simulink model "Data_Center_24hr_Total_Power_Analysis_Ref83_Simulation"  (R2024b)
settings: Solver=ode45  StartTime=0.0  StopTime=24  RelTol=1e-4
InitFcn:
  | load('DataCenterPower.mat')
libraries: spsThreePhaseSeriesRLCBranchLib x8, spsThreePhaseParallelRLCLoadLib x7, spsThreePhaseDynamicLoadLib x7, spsGroundLib x4, spsThreePhaseProgrammableVoltageSourceLib x2, spsThreePhaseTransformerTwoWindingsLib x2, spsThreePhaseBreakerLib x2, spsPower3phInstantaneousLib x1, spsThreePhaseVIMeasurementLib x1, sps_lib x1
settings Model: Creator=Kapla  LastModifiedBy=Kapla
settings DataIOCC: SaveFormat=Array  SaveOutput=off  SaveTime=off  ReturnWorkspaceOutputs=off
settings DebuggingCC: SaveWithParameterizedLinksMsg=none  IgnoredZcDiagnostic=none  StateNameClashWarn=warning  ArithmeticOperatorsInVariantConditions=warning
settings GRTTargetCC: TargetLangStandard=C89/C90 (ANSI)

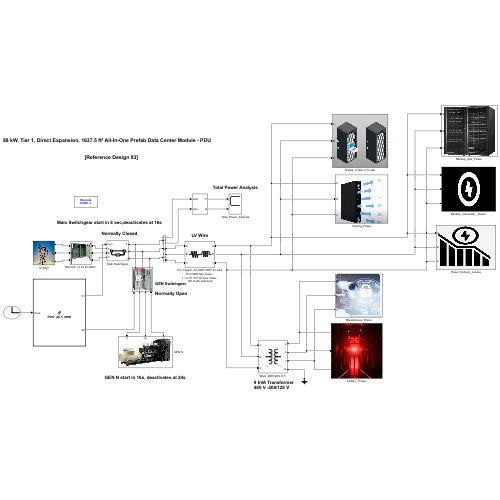
[thumbnail: Simulink's stored preview of the top-level diagram]
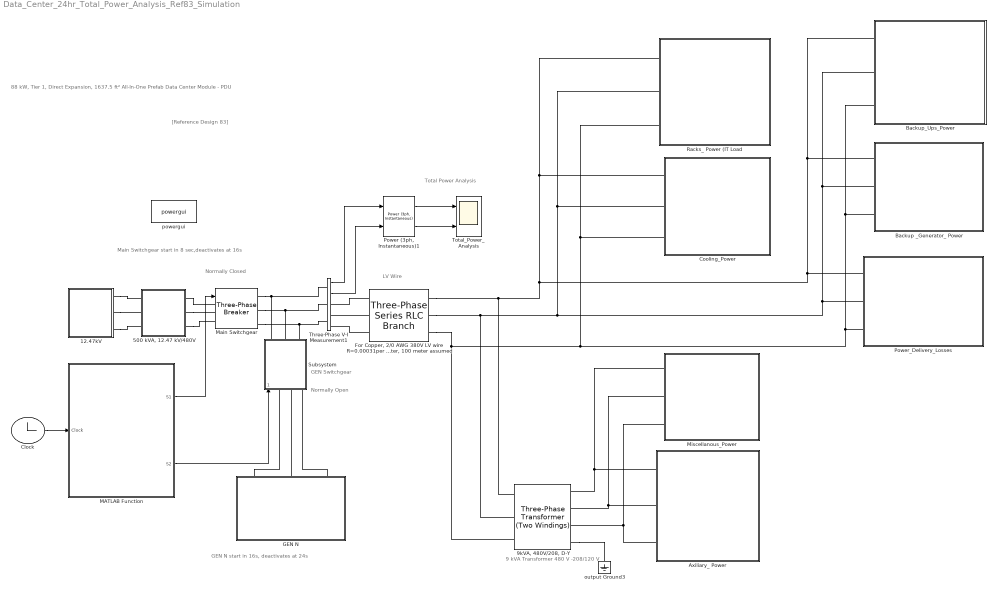
== system Data_Center_24hr_Total_Power_Analysis_Ref83_Simulation ==
  note: LV Wire
  note: Normally Open
  note: Normally Closed
  note: Main Switchgear start in 8 sec,deactivates at 16s
  note: GEN N start in 16s, deactivates at 24s
  note: GEN Switchgear
  note: [Reference Design 83]
  note: 88 kW, Tier 1, Direct Expansion, 1637.5 ft² All-In-One Prefab Data Center Module - PDU
  note: 9 kVA Transformer
      | 480 V -208/120 V
  note: Total Power Analysis
  12.47kV : Subsystem
      mask Display: image('Power_Grid_.png');
  "500 kVA, 12.47 kV/480V " : Subsystem
      mask Display: image('Data_Center_Transformer_Tier_1.png');
  "9kVA, 480V/208, D-Y" : spsThreePhaseTransformerTwoWindingsLib/Three-Phase Transformer (Two Windings)  Winding1Connection=Yg  Winding2Connection=Yn  CoreType=Three single-phase transformers  SetSaturation=off  Hysteresis=off  DataFile='hysteresis'  SetInitialFlux=off  Measurements=None  UNITS=pu  NominalPower=[ 9e3 , 60 ]  Winding1=[ 480 , 0.002 , 0.08 ]  Winding2=[ 208 , 0.002 , 0.08 ]  Rm=500  Lm=500  L0=0.5  Saturation=[ 0,0 ; 0.0024,1.2 ; 1.0,1.52 ]  InitialFluxes=[ 0.8 , -0.8 , 0.7 ]  BreakLoop=off  DiscreteSolver=Trapezoidal iterative  DataType=off  TransfoNumber=1
  Axiliary_ Power : Subsystem
      mask Display: image('Lighting_monitoring.png');
  "Backup _Generator_ Power " : Subsystem
      mask Display: image('back up_generator_power.png');
  "Backup_Ups_Power " : Subsystem
      mask Display: image('UPS.png');
  Clock : Clock
  Cooling_Power : Subsystem
      mask Display: image('Coolin.png');
  "For Copper, 2/0 AWG 380V LV wire R=0.00031per meter, L = 0.15 *10^-6 H per meter, 100 meter assumed " : spsThreePhaseSeriesRLCBranchLib/Three-Phase Series RLC Branch  LConnTagsString=A|B|C  RConnTagsString=A|B|C  BranchType=RL  Resistance=0.00031*100  Inductance=0.15e-6*100  Capacitance=[]  Measurements=None
  GEN N : Subsystem
      mask Display: image('Back_up_Generator.png');
  MATLAB Function : MATLAB Function  TreatAsAtomicUnit=on
  Main Switchgear : spsThreePhaseBreakerLib/Three-Phase Breaker  InitialState=closed  SwitchA=on  SwitchB=on  SwitchC=on  SwitchTimes="[8  16]"  External=on  BreakerResistance=10  SnubberResistance=1e-6  SnubberCapacitance=inf  Measurements=None
  Miscellanous_Power : Subsystem
      mask Display: image('Data_Center_Security.png');
  "Power (3ph, Instantaneous)1" : spsPower3phInstantaneousLib/Power (3ph, Instantaneous)
  Power_Delivery_Losses : Subsystem
      mask Display: image('Power_Delivery_losses.png');
  Racks_ Power (IT Load : Subsystem
      mask Display: image('racks_server.png');
  Subsystem : Subsystem
      mask Display: image('GEN_Switch_gear_500kW.png');
  Three-Phase V-I Measurement1 : spsThreePhaseVIMeasurementLib/Three-Phase V-I Measurement  VoltageMeasurement=phase-to-ground  SetLabelV=off  LabelV=V1  Vpu=off  VpuLL=off  CurrentMeasurement=yes  SetLabelI=off  LabelI=I1  Ipu=off  Pbase=100e6  Vbase=500e3  OutputType=Magnitude  PhasorSimulation=off  PSBequivalent=0
  Total_Power_Analysis : Scope  NumInputPorts=2
  output Ground3 : spsGroundLib/Ground  LConnTagsString=a
  powergui : sps_lib/powergui  Priority=1  SimulationMode=Discrete  SampleTime=100e-6  frequency=60  Iterations=50  frequencyindice=60  Pbase=100e6  ErrMax=1e-4  UnitsV=kV  UnitsW=MW  buscounter=0  FunctionMessages=off  echomessages=off  EnableUseOfTLC=off  CurrentSourceSwitches=off  DisableSnubberDevices=off  DisableRonSwitches=off  DisableVfSwitches=off  DisplayEquations=off  AutomaticDiscreteSolvers=off  SolverType=Tustin/Backward Euler (TBE)  Interpol=off  ExternalGateDelay=off  methode=off  Ts=100  x0status=blocks  SPID=on  SwTol=0  HookPort=off  NonlinearTolerance=1e-4  nMaxIteration=100  ContinueOnMaxIteration=off  RestoreLinks=warning  ResistiveCurrentMeasurement=off  Frange=[0:2:500]  Ylog=off  Xlog=on  ShowGrid=off  save=off  variable=ZData  structure=0  ZoomFFT=off  StartTime=0.0  cycles=1  DisplayStyle=1  fundamental=60  FreqAxis=off  MaxFrequency=1000  frequencyindicesteady=1  RmsSteady=1  display=off
  wires:
  Three-Phase V-I Measurement1/2 -> "Power (3ph, Instantaneous)1"/2
  Three-Phase V-I Measurement1/1 -> "Power (3ph, Instantaneous)1"/1
  MATLAB Function/1(S1) -> Main Switchgear/1
  Clock/1 -> MATLAB Function/1(Clock)
  "Power (3ph, Instantaneous)1"/1 -> Total_Power_Analysis/1
  "Power (3ph, Instantaneous)1"/2 -> Total_Power_Analysis/2
  MATLAB Function/2(S2) -> Subsystem/1(com)
  connections:
  Power_Delivery_Losses/LConn3 -- "9kVA, 480V/208, D-Y"/LConn3 -- "For Copper, 2/0 AWG 380V LV wire R=0.00031per meter, L = 0.15 *10^-6 H per meter, 100 meter assumed "/RConn3 -- Racks_ Power (IT Load/LConn3 -- Cooling_Power/LConn3 -- "Backup _Generator_ Power "/LConn3 -- "Backup_Ups_Power "/LConn3
  Power_Delivery_Losses/LConn2 -- "9kVA, 480V/208, D-Y"/LConn2 -- "For Copper, 2/0 AWG 380V LV wire R=0.00031per meter, L = 0.15 *10^-6 H per meter, 100 meter assumed "/RConn2 -- Racks_ Power (IT Load/LConn2 -- Cooling_Power/LConn2 -- "Backup _Generator_ Power "/LConn2 -- "Backup_Ups_Power "/LConn2
  Cooling_Power/LConn1 -- Racks_ Power (IT Load/LConn1 -- "9kVA, 480V/208, D-Y"/LConn1 -- "For Copper, 2/0 AWG 380V LV wire R=0.00031per meter, L = 0.15 *10^-6 H per meter, 100 meter assumed "/RConn1 -- "Backup_Ups_Power "/LConn1 -- "Backup _Generator_ Power "/LConn1 -- Power_Delivery_Losses/LConn1
  Axiliary_ Power/LConn1 -- Miscellanous_Power/LConn1 -- "9kVA, 480V/208, D-Y"/RConn1
  Axiliary_ Power/LConn3 -- Miscellanous_Power/LConn3 -- "9kVA, 480V/208, D-Y"/RConn3
  Axiliary_ Power/LConn2 -- Miscellanous_Power/LConn2 -- "9kVA, 480V/208, D-Y"/RConn2
  "9kVA, 480V/208, D-Y"/RConn4 -- output Ground3/LConn1
  Main Switchgear/RConn1 -- Subsystem/RConn1 -- Three-Phase V-I Measurement1/LConn1
  Main Switchgear/RConn2 -- Subsystem/RConn2 -- Three-Phase V-I Measurement1/LConn2
  Main Switchgear/RConn3 -- Subsystem/RConn3 -- Three-Phase V-I Measurement1/LConn3
  12.47kV/RConn1 -- "500 kVA, 12.47 kV/480V "/LConn1
  "500 kVA, 12.47 kV/480V "/RConn1 -- Main Switchgear/LConn1
  "500 kVA, 12.47 kV/480V "/RConn2 -- Main Switchgear/LConn2
  12.47kV/RConn2 -- "500 kVA, 12.47 kV/480V "/LConn2
  "500 kVA, 12.47 kV/480V "/RConn3 -- Main Switchgear/LConn3
  12.47kV/RConn3 -- "500 kVA, 12.47 kV/480V "/LConn3
  GEN N/RConn1 -- Subsystem/LConn1
  GEN N/RConn2 -- Subsystem/LConn2
  GEN N/RConn3 -- Subsystem/LConn3
  "For Copper, 2/0 AWG 380V LV wire R=0.00031per meter, L = 0.15 *10^-6 H per meter, 100 meter assumed "/LConn1 -- Three-Phase V-I Measurement1/RConn1
  "For Copper, 2/0 AWG 380V LV wire R=0.00031per meter, L = 0.15 *10^-6 H per meter, 100 meter assumed "/LConn2 -- Three-Phase V-I Measurement1/RConn2
  "For Copper, 2/0 AWG 380V LV wire R=0.00031per meter, L = 0.15 *10^-6 H per meter, 100 meter assumed "/LConn3 -- Three-Phase V-I Measurement1/RConn3

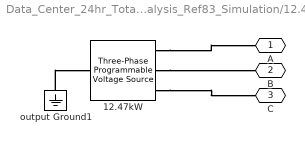
== system Data_Center_24hr_Total_Power_Analysis_Ref83_Simulation/12.47kV ==
  12.47kW : spsThreePhaseProgrammableVoltageSourceLib/Three-Phase Programmable Voltage Source  PositiveSequence="[12.47e3  0 60]"  VariationEntity=None  VariationType=Step  VariationTypeAlt=Step  VariationStep=-0.5  VariationRate=10  VariationMagnitude=0.5  VariationFrequency=1  VariationTiming=[0.2 1.2]  VariationPhaseA=off  Amplitudes=[1 0.8 1.2 1.0]  TimeValues=[0 0.1 0.15 0.2]  HarmonicGeneration=off  HarmonicA=[3 0.2 -25 0]  HarmonicB="[2 0.15  35 2]"  Timing="[0.05  3]"  BusType=swing  Pref=0  Qref=0  Qmin=-inf  Qmax=inf
  output Ground1 : spsGroundLib/Ground  LConnTagsString=a
  A : PMIOPort  Side=Right
  B : PMIOPort  Port=2  Side=Right
  C : PMIOPort  Port=3  Side=Right
  connections:
  output Ground1/LConn1 -- 12.47kW/LConn1
  12.47kW/RConn2 -- B/RConn1
  12.47kW/RConn3 -- C/RConn1
  12.47kW/RConn1 -- A/RConn1

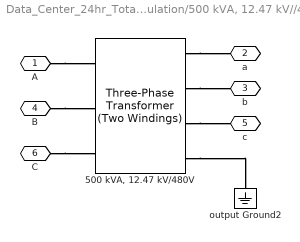
== system Data_Center_24hr_Total_Power_Analysis_Ref83_Simulation/500 kVA, 12.47 kV//480V  ==
  "500 kVA, 12.47 kV/480V " : spsThreePhaseTransformerTwoWindingsLib/Three-Phase Transformer (Two Windings)  Winding1Connection=Yg  Winding2Connection=Yn  CoreType=Three single-phase transformers  SetSaturation=off  Hysteresis=off  DataFile='hysteresis'  SetInitialFlux=off  Measurements=None  UNITS=pu  NominalPower=[ 500e3 , 60 ]  Winding1=[ 12.47e3 , 0.002 , 0.08 ]  Winding2=[ 480 , 0.002 , 0.08 ]  Rm=500  Lm=500  L0=0.5  Saturation=[ 0,0 ; 0.0024,1.2 ; 1.0,1.52 ]  InitialFluxes=[ 0.8 , -0.8 , 0.7 ]  BreakLoop=off  DiscreteSolver=Trapezoidal iterative  DataType=off  TransfoNumber=1
  output Ground2 : spsGroundLib/Ground  LConnTagsString=a
  A : PMIOPort  Side=Left
  a : PMIOPort  Port=2  Side=Right
  b : PMIOPort  Port=3  Side=Right
  B : PMIOPort  Port=4  Side=Left
  c : PMIOPort  Port=5  Side=Right
  C : PMIOPort  Port=6  Side=Left
  connections:
  "500 kVA, 12.47 kV/480V "/RConn4 -- output Ground2/LConn1
  C/RConn1 -- "500 kVA, 12.47 kV/480V "/LConn3
  A/RConn1 -- "500 kVA, 12.47 kV/480V "/LConn1
  "500 kVA, 12.47 kV/480V "/RConn3 -- c/RConn1
  B/RConn1 -- "500 kVA, 12.47 kV/480V "/LConn2
  "500 kVA, 12.47 kV/480V "/RConn1 -- a/RConn1
  "500 kVA, 12.47 kV/480V "/RConn2 -- b/RConn1

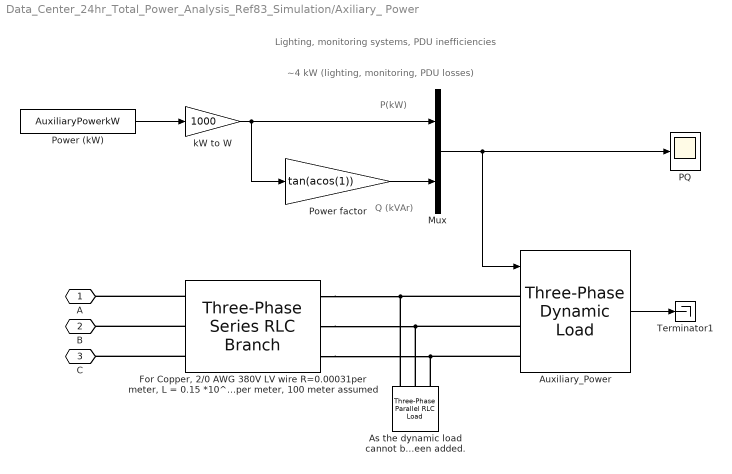
== system Data_Center_24hr_Total_Power_Analysis_Ref83_Simulation/Axiliary_ Power ==
  note: Q (kVAr)
  note: P(kW)
  note: ~4 kW (lighting, monitoring, PDU losses)
  note: Lighting, monitoring systems, PDU inefficiencies
  "As the dynamic load cannot be connected to an inductive network (R-L in series), a small resistive load (1 W) has been added." : spsThreePhaseParallelRLCLoadLib/Three-Phase Parallel RLC Load  LConnTagsString=A|B|C  Configuration=Y (grounded)  NominalVoltage=480  Vabc=[1e3 1e3 1e3]  Vabcp=[1e3 1e3 1e3]  NominalFrequency=60  UnbalancedPower=off  ActivePower=1  InductivePower=0  CapacitivePower=0  Pabc=[10e3 9e3 11e3]  QLabc=[100 90 110]  QCabc=[100 90 110]  Pabcp=[10e3 9e3 11e3]  QLabcp=[100 90 110]  QCabcp=[100 90 110]  Measurements=None  LoadType=constant Z
  Auxiliary_Power : spsThreePhaseDynamicLoadLib/Three-Phase Dynamic Load  NominalVoltage=[ 480 60 ]  ActiveReactivePowers=[3982 0*3982]  PositiveSequence=[1 -1.41063]  ExternalControl=on  NpNq="[1  1]"  TimeConstants="[0  0  0  0]"  MinimumVoltage=0.7  Tfilter=1e-4  LoadFlowParameters=[4 50000000 0 0 25000000]
  "For Copper, 2/0 AWG 380V LV wire R=0.00031per meter, L = 0.15 *10^-6 H per meter, 100 meter assumed " : spsThreePhaseSeriesRLCBranchLib/Three-Phase Series RLC Branch  LConnTagsString=A|B|C  RConnTagsString=A|B|C  BranchType=RL  Resistance=0.00031*100  Inductance=0.15e-6*100  Capacitance=[]  Measurements=None
  Mux : Mux  Inputs=2
  PQ : Scope
  Power (kW) : FromWorkspace  VariableName=AuxiliaryPowerkW
  Power factor : Gain  Gain=tan(acos(1))
  Terminator1 : Terminator
  kW to W : Gain  Gain=1000
  A : PMIOPort  Side=Left
  B : PMIOPort  Port=2  Side=Left
  C : PMIOPort  Port=3  Side=Left
  wires:
  Auxiliary_Power/1 -> Terminator1/1
  Power (kW)/1 -> kW to W/1
  kW to W/1 -> Power factor/1, Mux/1
  Power factor/1 -> Mux/2
  Mux/1 -> PQ/1, Auxiliary_Power/1
  connections:
  "For Copper, 2/0 AWG 380V LV wire R=0.00031per meter, L = 0.15 *10^-6 H per meter, 100 meter assumed "/LConn2 -- B/RConn1
  "For Copper, 2/0 AWG 380V LV wire R=0.00031per meter, L = 0.15 *10^-6 H per meter, 100 meter assumed "/LConn1 -- A/RConn1
  "For Copper, 2/0 AWG 380V LV wire R=0.00031per meter, L = 0.15 *10^-6 H per meter, 100 meter assumed "/LConn3 -- C/RConn1
  "For Copper, 2/0 AWG 380V LV wire R=0.00031per meter, L = 0.15 *10^-6 H per meter, 100 meter assumed "/RConn1 -- Auxiliary_Power/LConn1 -- "As the dynamic load cannot be connected to an inductive network (R-L in series), a small resistive load (1 W) has been added."/LConn1
  "For Copper, 2/0 AWG 380V LV wire R=0.00031per meter, L = 0.15 *10^-6 H per meter, 100 meter assumed "/RConn2 -- Auxiliary_Power/LConn2 -- "As the dynamic load cannot be connected to an inductive network (R-L in series), a small resistive load (1 W) has been added."/LConn2
  "For Copper, 2/0 AWG 380V LV wire R=0.00031per meter, L = 0.15 *10^-6 H per meter, 100 meter assumed "/RConn3 -- Auxiliary_Power/LConn3 -- "As the dynamic load cannot be connected to an inductive network (R-L in series), a small resistive load (1 W) has been added."/LConn3

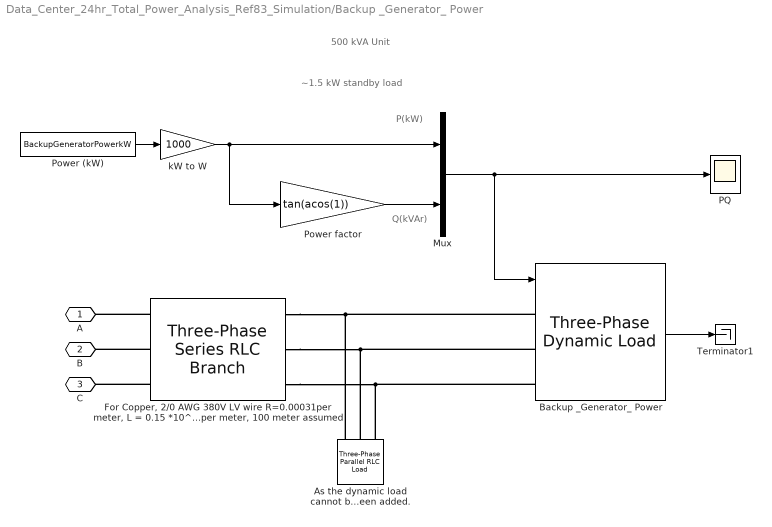
== system Data_Center_24hr_Total_Power_Analysis_Ref83_Simulation/Backup _Generator_ Power  ==
  note: Q(kVAr)
  note: P(kW)
  note: 500 kVA Unit
      |
      | ​
  note: ~1.5 kW standby load
      |
      | ​
  "As the dynamic load cannot be connected to an inductive network (R-L in series), a small resistive load (1 W) has been added." : spsThreePhaseParallelRLCLoadLib/Three-Phase Parallel RLC Load  LConnTagsString=A|B|C  Configuration=Y (grounded)  NominalVoltage=480  Vabc=[1e3 1e3 1e3]  Vabcp=[1e3 1e3 1e3]  NominalFrequency=60  UnbalancedPower=off  ActivePower=1  InductivePower=0  CapacitivePower=0  Pabc=[10e3 9e3 11e3]  QLabc=[100 90 110]  QCabc=[100 90 110]  Pabcp=[10e3 9e3 11e3]  QLabcp=[100 90 110]  QCabcp=[100 90 110]  Measurements=None  LoadType=constant Z
  "Backup _Generator_ Power " : spsThreePhaseDynamicLoadLib/Three-Phase Dynamic Load  NominalVoltage=[ 480 60 ]  ActiveReactivePowers=[1658 0*1658]  PositiveSequence=[1 -1.41063]  ExternalControl=on  NpNq="[1  1]"  TimeConstants="[0  0  0  0]"  MinimumVoltage=0.7  Tfilter=1e-4  LoadFlowParameters=[4 50000000 0 0 25000000]
  "For Copper, 2/0 AWG 380V LV wire R=0.00031per meter, L = 0.15 *10^-6 H per meter, 100 meter assumed " : spsThreePhaseSeriesRLCBranchLib/Three-Phase Series RLC Branch  LConnTagsString=A|B|C  RConnTagsString=A|B|C  BranchType=RL  Resistance=0.00031*100  Inductance=0.15e-6*100  Capacitance=[]  Measurements=None
  Mux : Mux  Inputs=2
  PQ : Scope
  Power (kW) : FromWorkspace  VariableName=BackupGeneratorPowerkW
  Power factor : Gain  Gain=tan(acos(1))
  Terminator1 : Terminator
  kW to W : Gain  Gain=1000
  A : PMIOPort  Side=Left
  B : PMIOPort  Port=2  Side=Left
  C : PMIOPort  Port=3  Side=Left
  wires:
  Power (kW)/1 -> kW to W/1
  "Backup _Generator_ Power "/1 -> Terminator1/1
  kW to W/1 -> Power factor/1, Mux/1
  Power factor/1 -> Mux/2
  Mux/1 -> PQ/1, "Backup _Generator_ Power "/1
  connections:
  "For Copper, 2/0 AWG 380V LV wire R=0.00031per meter, L = 0.15 *10^-6 H per meter, 100 meter assumed "/RConn3 -- "As the dynamic load cannot be connected to an inductive network (R-L in series), a small resistive load (1 W) has been added."/LConn3 -- "Backup _Generator_ Power "/LConn3
  "For Copper, 2/0 AWG 380V LV wire R=0.00031per meter, L = 0.15 *10^-6 H per meter, 100 meter assumed "/RConn1 -- "As the dynamic load cannot be connected to an inductive network (R-L in series), a small resistive load (1 W) has been added."/LConn1 -- "Backup _Generator_ Power "/LConn1
  "For Copper, 2/0 AWG 380V LV wire R=0.00031per meter, L = 0.15 *10^-6 H per meter, 100 meter assumed "/RConn2 -- "As the dynamic load cannot be connected to an inductive network (R-L in series), a small resistive load (1 W) has been added."/LConn2 -- "Backup _Generator_ Power "/LConn2
  "For Copper, 2/0 AWG 380V LV wire R=0.00031per meter, L = 0.15 *10^-6 H per meter, 100 meter assumed "/LConn2 -- B/RConn1
  "For Copper, 2/0 AWG 380V LV wire R=0.00031per meter, L = 0.15 *10^-6 H per meter, 100 meter assumed "/LConn3 -- C/RConn1
  "For Copper, 2/0 AWG 380V LV wire R=0.00031per meter, L = 0.15 *10^-6 H per meter, 100 meter assumed "/LConn1 -- A/RConn1

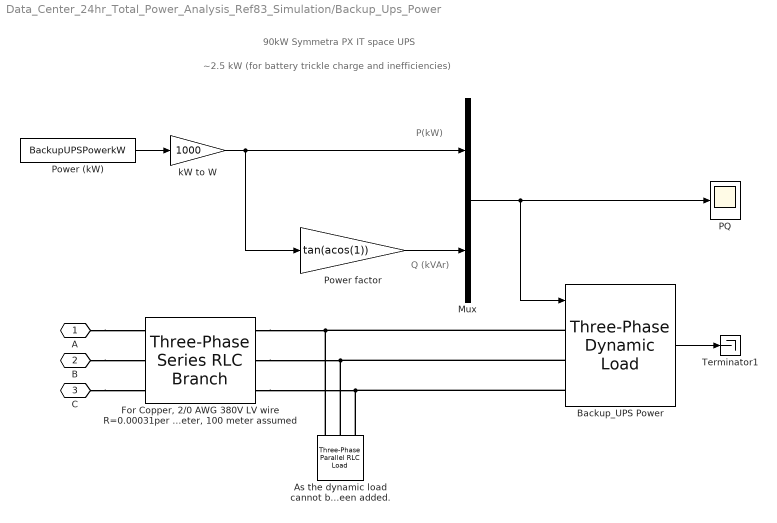
== system Data_Center_24hr_Total_Power_Analysis_Ref83_Simulation/Backup_Ups_Power  ==
  note: Q (kVAr)
  note: P(kW)
  note: ~2.5 kW (for battery trickle charge and inefficiencies)
  note: 90kW Symmetra PX IT space UPS
      |
      | ​
  "As the dynamic load cannot be connected to an inductive network (R-L in series), a small resistive load (1 W) has been added." : spsThreePhaseParallelRLCLoadLib/Three-Phase Parallel RLC Load  LConnTagsString=A|B|C  Configuration=Y (grounded)  NominalVoltage=480  Vabc=[1e3 1e3 1e3]  Vabcp=[1e3 1e3 1e3]  NominalFrequency=60  UnbalancedPower=off  ActivePower=1  InductivePower=0  CapacitivePower=0  Pabc=[10e3 9e3 11e3]  QLabc=[100 90 110]  QCabc=[100 90 110]  Pabcp=[10e3 9e3 11e3]  QLabcp=[100 90 110]  QCabcp=[100 90 110]  Measurements=None  LoadType=constant Z
  Backup_UPS Power : spsThreePhaseDynamicLoadLib/Three-Phase Dynamic Load  NominalVoltage=[ 480 60 ]  ActiveReactivePowers=[2559 0*2559]  PositiveSequence=[1 -1.41063]  ExternalControl=on  NpNq="[1  1]"  TimeConstants="[0  0  0  0]"  MinimumVoltage=0.7  Tfilter=1e-4  LoadFlowParameters=[4 50000000 0 0 25000000]
  "For Copper, 2/0 AWG 380V LV wire R=0.00031per meter, L = 0.15 *10^-6 H per meter, 100 meter assumed " : spsThreePhaseSeriesRLCBranchLib/Three-Phase Series RLC Branch  LConnTagsString=A|B|C  RConnTagsString=A|B|C  BranchType=RL  Resistance=0.00031*100  Inductance=0.15e-6*100  Capacitance=[]  Measurements=None
  Mux : Mux  Inputs=2
  PQ : Scope
  Power (kW) : FromWorkspace  VariableName=BackupUPSPowerkW
  Power factor : Gain  Gain=tan(acos(1))
  Terminator1 : Terminator
  kW to W : Gain  Gain=1000
  A : PMIOPort  Side=Left
  B : PMIOPort  Port=2  Side=Left
  C : PMIOPort  Port=3  Side=Left
  wires:
  Power (kW)/1 -> kW to W/1
  kW to W/1 -> Power factor/1, Mux/1
  Backup_UPS Power/1 -> Terminator1/1
  Power factor/1 -> Mux/2
  Mux/1 -> PQ/1, Backup_UPS Power/1
  connections:
  A/RConn1 -- "For Copper, 2/0 AWG 380V LV wire R=0.00031per meter, L = 0.15 *10^-6 H per meter, 100 meter assumed "/LConn1
  C/RConn1 -- "For Copper, 2/0 AWG 380V LV wire R=0.00031per meter, L = 0.15 *10^-6 H per meter, 100 meter assumed "/LConn3
  B/RConn1 -- "For Copper, 2/0 AWG 380V LV wire R=0.00031per meter, L = 0.15 *10^-6 H per meter, 100 meter assumed "/LConn2
  "For Copper, 2/0 AWG 380V LV wire R=0.00031per meter, L = 0.15 *10^-6 H per meter, 100 meter assumed "/RConn1 -- Backup_UPS Power/LConn1 -- "As the dynamic load cannot be connected to an inductive network (R-L in series), a small resistive load (1 W) has been added."/LConn1
  "For Copper, 2/0 AWG 380V LV wire R=0.00031per meter, L = 0.15 *10^-6 H per meter, 100 meter assumed "/RConn2 -- Backup_UPS Power/LConn2 -- "As the dynamic load cannot be connected to an inductive network (R-L in series), a small resistive load (1 W) has been added."/LConn2
  "For Copper, 2/0 AWG 380V LV wire R=0.00031per meter, L = 0.15 *10^-6 H per meter, 100 meter assumed "/RConn3 -- Backup_UPS Power/LConn3 -- "As the dynamic load cannot be connected to an inductive network (R-L in series), a small resistive load (1 W) has been added."/LConn3

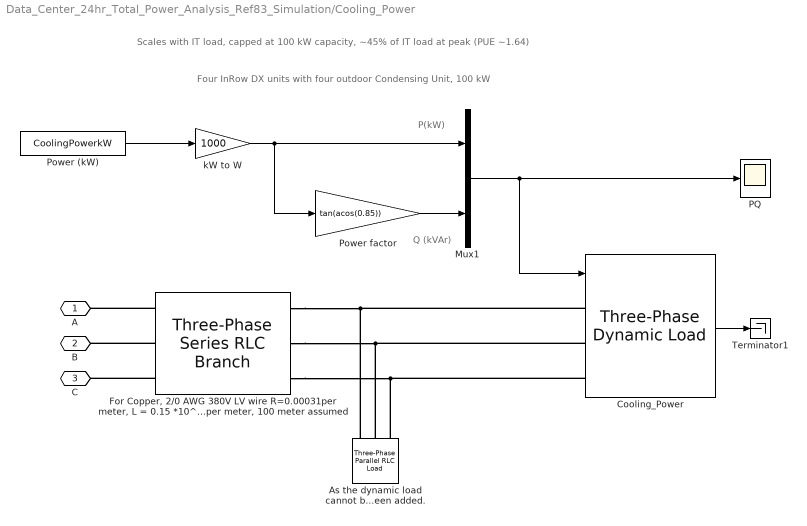
== system Data_Center_24hr_Total_Power_Analysis_Ref83_Simulation/Cooling_Power ==
  note: Q (kVAr)
  note: P(kW)
  note: Four InRow DX units with four outdoor Condensing Unit, 100 kW
  note: Scales with IT load, capped at 100 kW capacity, ~45% of IT load at peak (PUE ~1.64)
  "As the dynamic load cannot be connected to an inductive network (R-L in series), a small resistive load (1 W) has been added." : spsThreePhaseParallelRLCLoadLib/Three-Phase Parallel RLC Load  LConnTagsString=A|B|C  Configuration=Y (grounded)  NominalVoltage=480  Vabc=[1e3 1e3 1e3]  Vabcp=[1e3 1e3 1e3]  NominalFrequency=60  UnbalancedPower=off  ActivePower=1  InductivePower=0  CapacitivePower=0  Pabc=[10e3 9e3 11e3]  QLabc=[100 90 110]  QCabc=[100 90 110]  Pabcp=[10e3 9e3 11e3]  QLabcp=[100 90 110]  QCabcp=[100 90 110]  Measurements=None  LoadType=constant Z
  Cooling_Power : spsThreePhaseDynamicLoadLib/Three-Phase Dynamic Load  NominalVoltage=[ 480 60 ]  ActiveReactivePowers=[20378 0.61974*20378]  PositiveSequence=[1 -1.41063]  ExternalControl=on  NpNq="[1  1]"  TimeConstants="[0  0  0  0]"  MinimumVoltage=0.7  Tfilter=1e-4  LoadFlowParameters=[4 50000000 0 0 25000000]
  "For Copper, 2/0 AWG 380V LV wire R=0.00031per meter, L = 0.15 *10^-6 H per meter, 100 meter assumed " : spsThreePhaseSeriesRLCBranchLib/Three-Phase Series RLC Branch  LConnTagsString=A|B|C  RConnTagsString=A|B|C  BranchType=RL  Resistance=0.00031*100  Inductance=0.15e-6*100  Capacitance=[]  Measurements=None
  Mux1 : Mux  Inputs=2
  PQ : Scope
  Power (kW) : FromWorkspace  VariableName=CoolingPowerkW
  Power factor : Gain  Gain=tan(acos(0.85))
  Terminator1 : Terminator
  kW to W : Gain  Gain=1000
  A : PMIOPort  Side=Left
  B : PMIOPort  Port=2  Side=Left
  C : PMIOPort  Port=3  Side=Left
  wires:
  Power (kW)/1 -> kW to W/1
  Cooling_Power/1 -> Terminator1/1
  kW to W/1 -> Mux1/1, Power factor/1
  Power factor/1 -> Mux1/2
  Mux1/1 -> PQ/1, Cooling_Power/1
  connections:
  "For Copper, 2/0 AWG 380V LV wire R=0.00031per meter, L = 0.15 *10^-6 H per meter, 100 meter assumed "/LConn3 -- C/RConn1
  "For Copper, 2/0 AWG 380V LV wire R=0.00031per meter, L = 0.15 *10^-6 H per meter, 100 meter assumed "/LConn2 -- B/RConn1
  "For Copper, 2/0 AWG 380V LV wire R=0.00031per meter, L = 0.15 *10^-6 H per meter, 100 meter assumed "/LConn1 -- A/RConn1
  "For Copper, 2/0 AWG 380V LV wire R=0.00031per meter, L = 0.15 *10^-6 H per meter, 100 meter assumed "/RConn1 -- Cooling_Power/LConn1 -- "As the dynamic load cannot be connected to an inductive network (R-L in series), a small resistive load (1 W) has been added."/LConn1
  "For Copper, 2/0 AWG 380V LV wire R=0.00031per meter, L = 0.15 *10^-6 H per meter, 100 meter assumed "/RConn2 -- Cooling_Power/LConn2 -- "As the dynamic load cannot be connected to an inductive network (R-L in series), a small resistive load (1 W) has been added."/LConn2
  "For Copper, 2/0 AWG 380V LV wire R=0.00031per meter, L = 0.15 *10^-6 H per meter, 100 meter assumed "/RConn3 -- Cooling_Power/LConn3 -- "As the dynamic load cannot be connected to an inductive network (R-L in series), a small resistive load (1 W) has been added."/LConn3

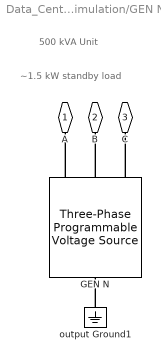
== system Data_Center_24hr_Total_Power_Analysis_Ref83_Simulation/GEN N ==
  note: ~1.5 kW standby load
      |
      | ​
  note: 500 kVA Unit
      |
      | ​
  GEN N : spsThreePhaseProgrammableVoltageSourceLib/Three-Phase Programmable Voltage Source  PositiveSequence="[480 0  60]"  VariationEntity=None  VariationType=Step  VariationTypeAlt=Step  VariationStep=-0.5  VariationRate=10  VariationMagnitude=0.5  VariationFrequency=1  VariationTiming=[0.2 1.2]  VariationPhaseA=off  Amplitudes=[1 0.8 1.2 1.0]  TimeValues=[0 0.1 0.15 0.2]  HarmonicGeneration=off  HarmonicA=[3 0.2 -25 0]  HarmonicB="[2 0.15  35 2]"  Timing="[0.05  3]"  BusType=PV  Pref=500e3  Qref=0  Qmin=-inf  Qmax=inf
  output Ground1 : spsGroundLib/Ground  LConnTagsString=a
  A : PMIOPort  Side=Right
  B : PMIOPort  Port=2  Side=Right
  C : PMIOPort  Port=3  Side=Right
  connections:
  GEN N/RConn2 -- B/RConn1
  output Ground1/LConn1 -- GEN N/LConn1
  GEN N/RConn1 -- A/RConn1
  GEN N/RConn3 -- C/RConn1

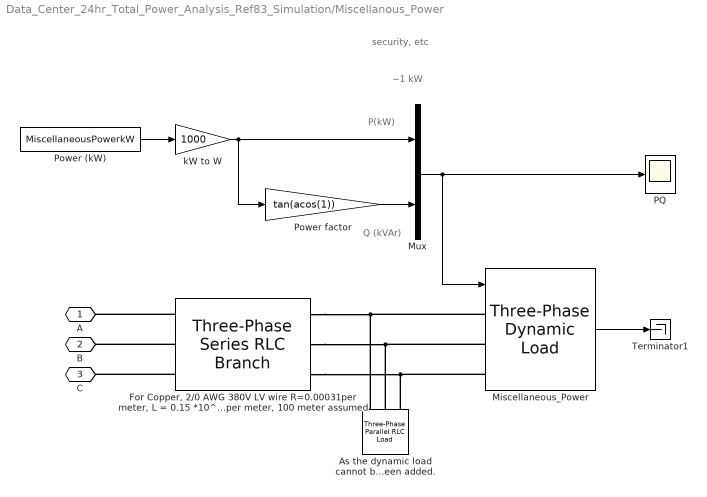
== system Data_Center_24hr_Total_Power_Analysis_Ref83_Simulation/Miscellanous_Power ==
  note: Q (kVAr)
  note: P(kW)
  note: security, etc
      |
      | ​
      |
      | ​
  note: ~1 kW
  "As the dynamic load cannot be connected to an inductive network (R-L in series), a small resistive load (1 W) has been added." : spsThreePhaseParallelRLCLoadLib/Three-Phase Parallel RLC Load  LConnTagsString=A|B|C  Configuration=Y (grounded)  NominalVoltage=480  Vabc=[1e3 1e3 1e3]  Vabcp=[1e3 1e3 1e3]  NominalFrequency=60  UnbalancedPower=off  ActivePower=1  InductivePower=0  CapacitivePower=0  Pabc=[10e3 9e3 11e3]  QLabc=[100 90 110]  QCabc=[100 90 110]  Pabcp=[10e3 9e3 11e3]  QLabcp=[100 90 110]  QCabcp=[100 90 110]  Measurements=None  LoadType=constant Z
  "For Copper, 2/0 AWG 380V LV wire R=0.00031per meter, L = 0.15 *10^-6 H per meter, 100 meter assumed " : spsThreePhaseSeriesRLCBranchLib/Three-Phase Series RLC Branch  LConnTagsString=A|B|C  RConnTagsString=A|B|C  BranchType=RL  Resistance=0.00031*100  Inductance=0.15e-6*100  Capacitance=[]  Measurements=None
  Miscellaneous_Power : spsThreePhaseDynamicLoadLib/Three-Phase Dynamic Load  NominalVoltage=[ 480 60 ]  ActiveReactivePowers=[1052 0*1052]  PositiveSequence=[1 -1.41063]  ExternalControl=on  NpNq="[1  1]"  TimeConstants="[0  0  0  0]"  MinimumVoltage=0.7  Tfilter=1e-4  LoadFlowParameters=[4 50000000 0 0 25000000]
  Mux : Mux  Inputs=2
  PQ : Scope
  Power (kW) : FromWorkspace  VariableName=MiscellaneousPowerkW
  Power factor : Gain  Gain=tan(acos(1))
  Terminator1 : Terminator
  kW to W : Gain  Gain=1000
  A : PMIOPort  Side=Left
  B : PMIOPort  Port=2  Side=Left
  C : PMIOPort  Port=3  Side=Left
  wires:
  Power (kW)/1 -> kW to W/1
  Miscellaneous_Power/1 -> Terminator1/1
  kW to W/1 -> Mux/1, Power factor/1
  Mux/1 -> PQ/1, Miscellaneous_Power/1
  Power factor/1 -> Mux/2
  connections:
  "For Copper, 2/0 AWG 380V LV wire R=0.00031per meter, L = 0.15 *10^-6 H per meter, 100 meter assumed "/LConn2 -- B/RConn1
  "For Copper, 2/0 AWG 380V LV wire R=0.00031per meter, L = 0.15 *10^-6 H per meter, 100 meter assumed "/LConn1 -- A/RConn1
  "For Copper, 2/0 AWG 380V LV wire R=0.00031per meter, L = 0.15 *10^-6 H per meter, 100 meter assumed "/LConn3 -- C/RConn1
  Miscellaneous_Power/LConn1 -- "For Copper, 2/0 AWG 380V LV wire R=0.00031per meter, L = 0.15 *10^-6 H per meter, 100 meter assumed "/RConn1 -- "As the dynamic load cannot be connected to an inductive network (R-L in series), a small resistive load (1 W) has been added."/LConn1
  Miscellaneous_Power/LConn2 -- "For Copper, 2/0 AWG 380V LV wire R=0.00031per meter, L = 0.15 *10^-6 H per meter, 100 meter assumed "/RConn2 -- "As the dynamic load cannot be connected to an inductive network (R-L in series), a small resistive load (1 W) has been added."/LConn2
  Miscellaneous_Power/LConn3 -- "For Copper, 2/0 AWG 380V LV wire R=0.00031per meter, L = 0.15 *10^-6 H per meter, 100 meter assumed "/RConn3 -- "As the dynamic load cannot be connected to an inductive network (R-L in series), a small resistive load (1 W) has been added."/LConn3

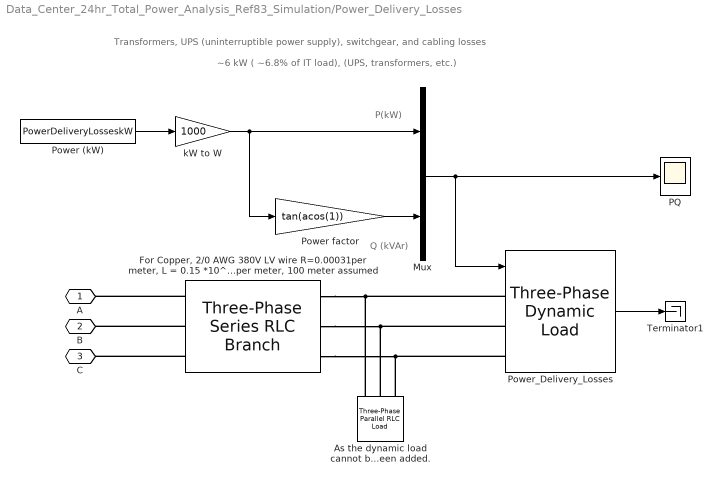
== system Data_Center_24hr_Total_Power_Analysis_Ref83_Simulation/Power_Delivery_Losses ==
  note: Q (kVAr)
  note: P(kW)
  note: ~6 kW ( ~6.8% of IT load), (UPS, transformers, etc.)
  note: Transformers, UPS (uninterruptible power supply), switchgear, and cabling losses
  "As the dynamic load cannot be connected to an inductive network (R-L in series), a small resistive load (1 W) has been added." : spsThreePhaseParallelRLCLoadLib/Three-Phase Parallel RLC Load  LConnTagsString=A|B|C  Configuration=Y (grounded)  NominalVoltage=480  Vabc=[1e3 1e3 1e3]  Vabcp=[1e3 1e3 1e3]  NominalFrequency=60  UnbalancedPower=off  ActivePower=1  InductivePower=0  CapacitivePower=0  Pabc=[10e3 9e3 11e3]  QLabc=[100 90 110]  QCabc=[100 90 110]  Pabcp=[10e3 9e3 11e3]  QLabcp=[100 90 110]  QCabcp=[100 90 110]  Measurements=None  LoadType=constant Z
  "For Copper, 2/0 AWG 380V LV wire R=0.00031per meter, L = 0.15 *10^-6 H per meter, 100 meter assumed " : spsThreePhaseSeriesRLCBranchLib/Three-Phase Series RLC Branch  LConnTagsString=A|B|C  RConnTagsString=A|B|C  BranchType=RL  Resistance=0.00031*100  Inductance=0.15e-6*100  Capacitance=[]  Measurements=None
  Mux : Mux  Inputs=2
  PQ : Scope
  Power (kW) : FromWorkspace  VariableName=PowerDeliveryLosseskW
  Power factor : Gain  Gain=tan(acos(1))
  Power_Delivery_Losses : spsThreePhaseDynamicLoadLib/Three-Phase Dynamic Load  NominalVoltage=[ 480 60 ]  ActiveReactivePowers=[3231 0*3231]  PositiveSequence=[1 -1.41063]  ExternalControl=on  NpNq="[1  1]"  TimeConstants="[0  0  0  0]"  MinimumVoltage=0.7  Tfilter=1e-4  LoadFlowParameters=[4 50000000 0 0 25000000]
  Terminator1 : Terminator
  kW to W : Gain  Gain=1000
  A : PMIOPort  Side=Left
  B : PMIOPort  Port=2  Side=Left
  C : PMIOPort  Port=3  Side=Left
  wires:
  Power_Delivery_Losses/1 -> Terminator1/1
  Power (kW)/1 -> kW to W/1
  kW to W/1 -> Power factor/1, Mux/1
  Mux/1 -> Power_Delivery_Losses/1, PQ/1
  Power factor/1 -> Mux/2
  connections:
  "For Copper, 2/0 AWG 380V LV wire R=0.00031per meter, L = 0.15 *10^-6 H per meter, 100 meter assumed "/LConn3 -- C/RConn1
  "For Copper, 2/0 AWG 380V LV wire R=0.00031per meter, L = 0.15 *10^-6 H per meter, 100 meter assumed "/LConn1 -- A/RConn1
  "For Copper, 2/0 AWG 380V LV wire R=0.00031per meter, L = 0.15 *10^-6 H per meter, 100 meter assumed "/LConn2 -- B/RConn1
  "For Copper, 2/0 AWG 380V LV wire R=0.00031per meter, L = 0.15 *10^-6 H per meter, 100 meter assumed "/RConn1 -- Power_Delivery_Losses/LConn1 -- "As the dynamic load cannot be connected to an inductive network (R-L in series), a small resistive load (1 W) has been added."/LConn1
  "For Copper, 2/0 AWG 380V LV wire R=0.00031per meter, L = 0.15 *10^-6 H per meter, 100 meter assumed "/RConn2 -- Power_Delivery_Losses/LConn2 -- "As the dynamic load cannot be connected to an inductive network (R-L in series), a small resistive load (1 W) has been added."/LConn2
  "For Copper, 2/0 AWG 380V LV wire R=0.00031per meter, L = 0.15 *10^-6 H per meter, 100 meter assumed "/RConn3 -- Power_Delivery_Losses/LConn3 -- "As the dynamic load cannot be connected to an inductive network (R-L in series), a small resistive load (1 W) has been added."/LConn3

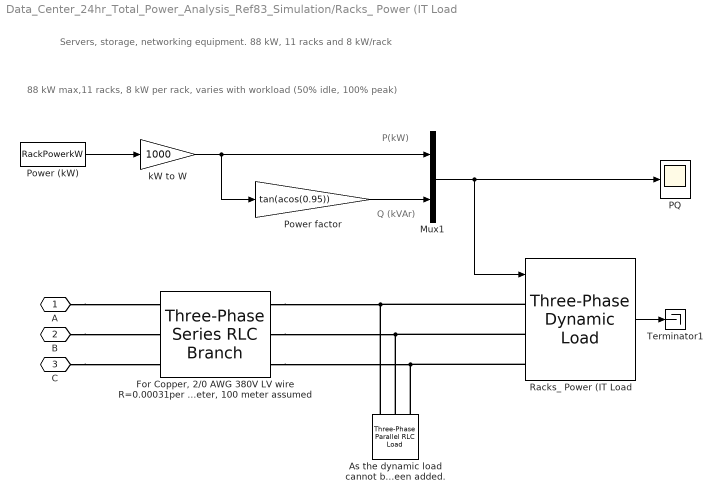
== system Data_Center_24hr_Total_Power_Analysis_Ref83_Simulation/Racks_ Power (IT Load ==
  note: Q (kVAr)
  note: Servers, storage, networking equipment. 88 kW, 11 racks and 8 kW/rack
  note: 88 kW max,11 racks, 8 kW per rack, varies with workload (50% idle, 100% peak)
  note: P(kW)
  "As the dynamic load cannot be connected to an inductive network (R-L in series), a small resistive load (1 W) has been added." : spsThreePhaseParallelRLCLoadLib/Three-Phase Parallel RLC Load  LConnTagsString=A|B|C  Configuration=Y (grounded)  NominalVoltage=480  Vabc=[1e3 1e3 1e3]  Vabcp=[1e3 1e3 1e3]  NominalFrequency=60  UnbalancedPower=off  ActivePower=1  InductivePower=0  CapacitivePower=0  Pabc=[10e3 9e3 11e3]  QLabc=[100 90 110]  QCabc=[100 90 110]  Pabcp=[10e3 9e3 11e3]  QLabcp=[100 90 110]  QCabcp=[100 90 110]  Measurements=None  LoadType=constant Z
  "For Copper, 2/0 AWG 380V LV wire R=0.00031per meter, L = 0.15 *10^-6 H per meter, 100 meter assumed " : spsThreePhaseSeriesRLCBranchLib/Three-Phase Series RLC Branch  LConnTagsString=A|B|C  RConnTagsString=A|B|C  BranchType=RL  Resistance=0.00031*100  Inductance=0.15e-6*100  Capacitance=[]  Measurements=None
  Mux1 : Mux  Inputs=2
  PQ : Scope
  Power (kW) : FromWorkspace  VariableName=RackPowerkW
  Power factor : Gain  Gain=tan(acos(0.95))
  Racks_ Power (IT Load : spsThreePhaseDynamicLoadLib/Three-Phase Dynamic Load  NominalVoltage=[ 480 60 ]  ActiveReactivePowers=[44993 0.32868*44993]  PositiveSequence=[1 -1.41063]  ExternalControl=on  NpNq="[1  1]"  TimeConstants="[0  0  0  0]"  MinimumVoltage=0.7  Tfilter=1e-4  LoadFlowParameters=[4 50000000 0 0 25000000]
  Terminator1 : Terminator
  kW to W : Gain  Gain=1000
  A : PMIOPort  Side=Left
  B : PMIOPort  Port=2  Side=Left
  C : PMIOPort  Port=3  Side=Left
  wires:
  Racks_ Power (IT Load/1 -> Terminator1/1
  Power (kW)/1 -> kW to W/1
  kW to W/1 -> Mux1/1, Power factor/1
  Power factor/1 -> Mux1/2
  Mux1/1 -> PQ/1, Racks_ Power (IT Load/1
  connections:
  C/RConn1 -- "For Copper, 2/0 AWG 380V LV wire R=0.00031per meter, L = 0.15 *10^-6 H per meter, 100 meter assumed "/LConn3
  B/RConn1 -- "For Copper, 2/0 AWG 380V LV wire R=0.00031per meter, L = 0.15 *10^-6 H per meter, 100 meter assumed "/LConn2
  A/RConn1 -- "For Copper, 2/0 AWG 380V LV wire R=0.00031per meter, L = 0.15 *10^-6 H per meter, 100 meter assumed "/LConn1
  "For Copper, 2/0 AWG 380V LV wire R=0.00031per meter, L = 0.15 *10^-6 H per meter, 100 meter assumed "/RConn1 -- Racks_ Power (IT Load/LConn1 -- "As the dynamic load cannot be connected to an inductive network (R-L in series), a small resistive load (1 W) has been added."/LConn1
  "For Copper, 2/0 AWG 380V LV wire R=0.00031per meter, L = 0.15 *10^-6 H per meter, 100 meter assumed "/RConn2 -- Racks_ Power (IT Load/LConn2 -- "As the dynamic load cannot be connected to an inductive network (R-L in series), a small resistive load (1 W) has been added."/LConn2
  "For Copper, 2/0 AWG 380V LV wire R=0.00031per meter, L = 0.15 *10^-6 H per meter, 100 meter assumed "/RConn3 -- Racks_ Power (IT Load/LConn3 -- "As the dynamic load cannot be connected to an inductive network (R-L in series), a small resistive load (1 W) has been added."/LConn3

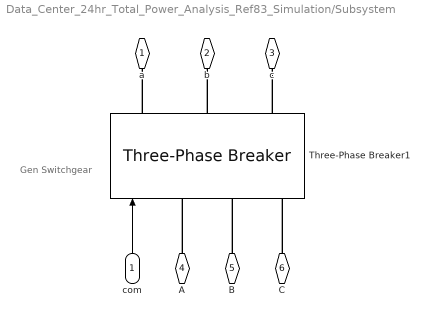
== system Data_Center_24hr_Total_Power_Analysis_Ref83_Simulation/Subsystem ==
  note: Gen Switchgear
  com : Inport
  Three-Phase Breaker1 : spsThreePhaseBreakerLib/Three-Phase Breaker  InitialState=open  SwitchA=on  SwitchB=on  SwitchC=on  SwitchTimes="[16  24]"  External=on  BreakerResistance=10  SnubberResistance=1e-6  SnubberCapacitance=inf  Measurements=None
  a : PMIOPort  Side=Right
  b : PMIOPort  Port=2  Side=Right
  c : PMIOPort  Port=3  Side=Right
  A : PMIOPort  Port=4  Side=Left
  B : PMIOPort  Port=5  Side=Left
  C : PMIOPort  Port=6  Side=Left
  wires:
  com/1 -> Three-Phase Breaker1/1
  connections:
  Three-Phase Breaker1/RConn3 -- c/RConn1
  Three-Phase Breaker1/RConn2 -- b/RConn1
  Three-Phase Breaker1/RConn1 -- a/RConn1
  A/RConn1 -- Three-Phase Breaker1/LConn1
  C/RConn1 -- Three-Phase Breaker1/LConn3
  B/RConn1 -- Three-Phase Breaker1/LConn2

== matlab function Data_Center_24hr_Total_Power_Analysis_Ref83_Simulation/MATLAB Function ==
  data: Clock input; S1 output; S2 output
function [S1, S2] = SwitchgearControl(Clock)
% SwitchgearControl - Determines the switchgear state based on clock time.
%
% Time intervals:
%  * Normal Operation:      0 <= Clock < 8  sec =>S1 =  1, S2 = 0 
%  * Grid Interruption:     8 <= Clock < 16 sec =>S1 =  0, S2 = 1
%  * Grid Restored:         16<= Clock <=24 sec =>S1 =  0, S2 = 0

T1 = 0;
T2 = 8;
T3 = 16;
T4 = 24;

if Clock >= T1 && Clock < T2
    % Normal Operation
    S1 = 1;
    S2 = 0;
elseif Clock >= T2 && Clock < T3
    % Grid Interruption
    S1 = 0;
    S2 = 1;
elseif Clock >= T3 && Clock <= T4
    % Grid Restored
    S1 = 0;
    S2 = 0;
else
    % Default state for times outside the defined intervals
    S1 = 0;
    S2 = 0;
end

end
